simulink model "bai_lam_lai"  (R2018a)
settings: Solver=VariableStepAuto  StartTime=0.0  StopTime=15  RelTol=1e-3
values from neighbouring files (symbols this model uses):
  km = 0.5    [Parameters.m]    (also in Parameters.mat; parametersAcc.m; parametersPos.m; parametersVel.m)
  KP = 5    [Parameters.m]    (also in Parameters.mat; parametersAcc.m = 26; parametersPos.m; parametersVel.m)
  Tm = 0    [Parameters.m]    (also in Parameters.mat = 5; parametersAcc.m = 0.025; parametersPos.m = 0.025; parametersVel.m = 0.025)
  TP = 0    [Parameters.m]    (also in Parameters.mat = 5; parametersAcc.m = 2.5; parametersPos.m = 2.5; parametersVel.m = 2.5)
settings Model: Creator=Nguyen Mai  LastModifiedBy=Nguyen Mai

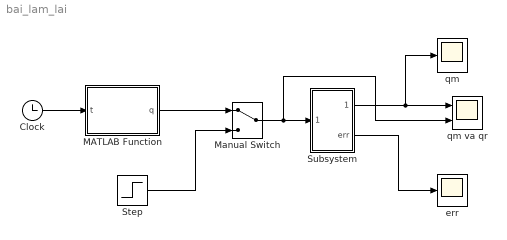
== system bai_lam_lai ==
  Clock : Clock
  MATLAB Function : MATLAB Function  TreatAsAtomicUnit=on
  Manual Switch : ManualSwitch
  Step : Step  SampleTime=0
  Subsystem : Subsystem
  err : Scope
  "qm " : Scope
  qm va qr : Scope  NumInputPorts=2
  wires:
  Clock/1 -> MATLAB Function/1(t)
  Step/1 -> Manual Switch/2
  Manual Switch/1 -> qm va qr/2, Subsystem/1(In1)
  Subsystem/1(qm) -> qm va qr/1, "qm "/1
  Subsystem/2(err) -> err/1
  MATLAB Function/1(q) -> Manual Switch/1

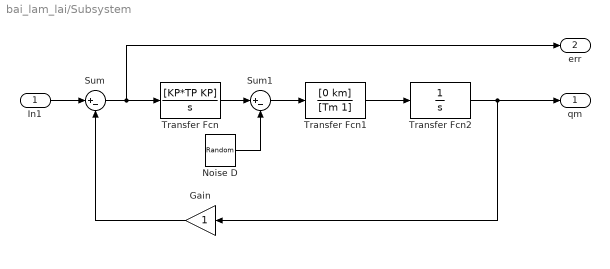
== system bai_lam_lai/Subsystem ==
  In1 : Inport
  Gain : Gain
  Noise D : UniformRandomNumber  Minimum=-0.01  Maximum=0.01  Seed=24  SampleTime=0.01
  Sum : Sum  Inputs=|+-
  Sum1 : Sum  Inputs=|+-
  Transfer Fcn : TransferFcn  Numerator=[KP*TP KP]  Denominator=[1 0]
  Transfer Fcn1 : TransferFcn  Numerator=[0 km]  Denominator=[Tm 1]
  Transfer Fcn2 : TransferFcn  Denominator=[1 0]
  qm : Outport
  err : Outport  Port=2
  wires:
  Transfer Fcn1/1 -> Transfer Fcn2/1
  Noise D/1 -> Sum1/2
  Sum/1 -> err/1, Transfer Fcn/1
  Transfer Fcn2/1 -> qm/1, Gain/1
  Sum1/1 -> Transfer Fcn1/1
  Transfer Fcn/1 -> Sum1/1
  Gain/1 -> Sum/2
  In1/1 -> Sum/1

== matlab function bai_lam_lai/MATLAB Function ==
  data: t input; q output
function q = fcn(t)
t0=0;
tf=40;
tc=4/5;
if t<tc
q=40+(125/8)*t^2;
else
if t<tf-tc
q=30+25*t;
else
q=1020-(125/8)*(40-t)^2;
end
end
